simulink model "example"  (R2016b)
settings: Solver=FixedStepAuto  StartTime=0.0  StopTime=10  FixedStep=0.001  RelTol=1e-3
undefined symbols (not defined in the file): a, b, c
libraries: simulink x1, blender x1
settings Model: Creator=GOD  LastModifiedBy=GOD

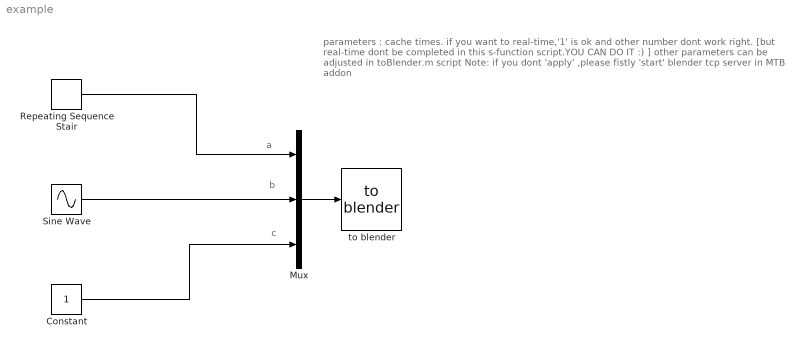
== system example ==
  note: parameters :
      | cache times. if you want to real-time,'1' is ok and other number dont work right.
      | [but real-time dont be completed in this s-function script.YOU CAN DO IT :) ]
      |
      | other parameters can be adjusted in toBlender.m script
      |
      | Note:
      | if you dont 'apply' ,please fistly 'start' blender tcp server in MTB addon
  note: c
  note: b
  note: a
  Constant : Constant
  Mux : Mux  Inputs=3
  Repeating Sequence Stair : simulink/Sources/Repeating Sequence Stair  OutValues=[3 1 4 2 1].'  tsamp=-1  OutMin=[]  OutMax=[]  OutDataTypeStr=double  OutputDataTypeScalingMode=double  OutDataType=fixdt(0,8)  ConRadixGroup=Best Precision: Vector-wise  OutScaling=2^-12
  Sine Wave : Sin  Frequency=10  SampleTime=0
  to blender : blender/to blender  host=127.0.0.1  port=20208  cachetimes=4  names=a,b,c
  wires:
  Sine Wave/1 -> Mux/2
  Repeating Sequence Stair/1 -> Mux/1
  Mux/1 -> to blender/1
  Constant/1 -> Mux/3
